simulink library "lib_FDM"  (R2019b)
settings: Solver=VariableStepAuto  StartTime=0.0  StopTime=10.0  RelTol=1e-3
values from neighbouring files (symbols this model uses):
  d = config.d_m    [computeTF.m]
undefined symbols (not defined in the file or in its folder): c_b_WGS, c_flat, c_grav, c_rot, c_rsma, Cd0, Cdcl, Cdcl2, Cl0, Cla, Cld, Cma, Cmd, Cmq, Cnb, Cnd, Cnr, Cra, Crd, Crp, Cy0, Cyb, Cyd, dmdt, Earth, HIL_Data, InitThrust, launchPos, me, mf, mp, Sref, tb, TF, theta0, WGS84
libraries: simulink_extras x14, $bdroot x7, simulink x5, lib_Fin_Deflections x3, aerolibasang x2, sharedtransform x1, aerolibtransform2 x1, aerolibbdyn x1, aerolibatmos2 x1, aerolibutil x1, aerolib6dof2 x1
(part 5 of 8)

== system lib_FDM/FDM/FDM_Sophisticated/stream_flow/calc_stream_flow/Subsystem1 ==
  vWEB : Inport
  vBEB : Inport  Port=2
  wBIB : Inport  Port=3
  rho : Inport  Port=4
  sos : Inport  Port=5
  AoA_Sideslip_Alphatot_Phi : Subsystem
      mask help:
      | Aus den Komponenten der Geschwindigkeit im ECEF-System, dargestellt im Body-System vBEB
      | werden Anstellwinkel (alpha), Schiebewinkel (beta), totaler Anstellwinkel (alpha_T) sowie Rollwinkel (phi) berechnet.
      | Die Ausgabe erfolgt als Bus in [rad]
      mask Help:
      | Name:
      | 
      |    AoA_sideslip_alphatot_phi
      | 
      | Beschreibung:
      | 
      |   Dieser Block berechnet Anstellwinkel, Schiebewinkel, totalen Anstellwinkel und Rollwinkel in [rad]
      |   aus der Geschwindigkeit vBEB (ECEF-System dargestellt in Body-Koordinaten)
      | 
      | Inputs   [dimension]  [data type] [unit]:
      | 
      |     vBEB    [3] [double] [m/s]
      | 
      | Outputs  [dimension]  [data type] [unit]:
      | 
      | aero_angle_bus [4] [bus] [-]
      |     alpha     [1] [double] [rad]
      |     beta       [1] [double] [rad]
      |     alpha_T [1] [double] [rad]
      |     phi         [1] [double] [rad]
      mask Display:
      | %port_label('input', 1, 'vBEB')
      | %port_label('output', 1, 'aero_angles')
      | disp('vBEB \rightarrow \alpha \beta \alpha_T \phi','texmode','on')
  Bus Selector : BusSelector  OutputSignals=al,be,th,fi
  Constant : Constant  Value=0.5
  Divide : Product  Inputs=*/
  Math Function1 : Math  Operator=square  SaturateOnIntegerOverflow=on
  Product1 : Product  Inputs=3
  Subtract : Sum  Inputs=+-
  calc_nondimensional_rates : Subsystem
  norm_of_vector : Subsystem
      mask help: computes the norm of a vector
      mask Help:
      | Name:
      | 
      |     norm_of_vector
      | 
      | Description:
      | 
      |     This block computes the L2-norm (length) of a vector.
      | 
      | Inputs  [size] [data type] [unit]:
      | 
      |     vector  [3] [double] [-]
      | 
      | Outputs  [size] [data type] [unit]:
      | 
      |     norm of vector  [1] [double] [-]
      mask Display: disp (' norm(r) ')
  al : Outport  VectorParamsAs1DForOutWhenUnconnected=off
  be : Outport  Port=2  VectorParamsAs1DForOutWhenUnconnected=off
  qdynB : Outport  Port=3  VectorParamsAs1DForOutWhenUnconnected=off
  MaB : Outport  Port=4  VectorParamsAs1DForOutWhenUnconnected=off
  a_vB : Outport  Port=5  VectorParamsAs1DForOutWhenUnconnected=off
  wBIB_star : Outport  Port=6  VectorParamsAs1DForOutWhenUnconnected=off
  th : Outport  Port=7  VectorParamsAs1DForOutWhenUnconnected=off
  fi : Outport  Port=8  VectorParamsAs1DForOutWhenUnconnected=off
  wires:
  Subtract/1 -> AoA_Sideslip_Alphatot_Phi/1(vBEB), norm_of_vector/1(vector)  "vBEB_a"
  vWEB/1 -> Subtract/2
  Bus Selector/4 -> fi/1  "<fi>"
  Bus Selector/3 -> th/1  "<th>"
  calc_nondimensional_rates/1(wBIB_star) -> wBIB_star/1
  wBIB/1 -> calc_nondimensional_rates/2(wBIB)
  Bus Selector/1 -> al/1  "<al>"
  rho/1 -> Product1/3
  Bus Selector/2 -> be/1  "<be>"
  Divide/1 -> MaB/1  "MaB"
  Constant/1 -> Product1/2
  Math Function1/1 -> Product1/1
  Product1/1 -> qdynB/1  "qdynB"
  norm_of_vector/1(norm_of_vector) -> Divide/1, a_vB/1, calc_nondimensional_rates/1(a_vB), Math Function1/1  "a_vB"
  vBEB/1 -> Subtract/1
  AoA_Sideslip_Alphatot_Phi/1(aero_angles) -> Bus Selector/1
  sos/1 -> Divide/2

== system lib_FDM/FDM/FDM_Sophisticated/stream_flow/calc_stream_flow/velocity_vector_transformation ==
  wIEE : Inport
  TIE : Inport  Port=2
  vBII : Inport  Port=3
  pBII : Inport  Port=4
  Add : Sum  Inputs=+-
  Product : Product  Multiplication=Matrix(*)
  cross_product : Subsystem
      mask help: cross product r3 = r1 x r2
      mask Help:
      | Name:
      | 
      |     cross_product
      | 
      | Description:
      | 
      |     This block implements the cross product r3 = r1 x r2.
      | 
      | Inputs  [size] [data type] [unit]:
      | 
      |     vector 1  [3] [double] [-]
      |     vector 2  [3] [double] [-]
      | 
      | Outputs  [size] [data type] [unit]:
      | 
      |     resulting vector  [3] [double] [-]
      mask Display: disp(' r3 = r1 x r2')
  vBEI : Outport  VectorParamsAs1DForOutWhenUnconnected=off
  wires:
  Add/1 -> vBEI/1  "vBEI"
  vBII/1 -> Add/1
  cross_product/1(r1_x_r2) -> Add/2  "de_vBEI"
  pBII/1 -> cross_product/2(r2)
  Product/1 -> cross_product/1(r1)  "wIEI"
  wIEE/1 -> Product/2
  TIE/1 -> Product/1

== system lib_FDM/FDM/FDM_Sophisticated/tmp/weather/atm_dynamic ==
  Add : Sum
  Add1 : Sum
  Bus Creator : BusCreator  Inputs=1
  Constant1 : Constant  Value=0
  Vector Concatenate : Concatenate  NumInputs=3
  course_angle_uncertainty : Constant  Value=HIL_Data.FDM.soph.bus1.unc_chW_bl
  course_angle_wind : Constant  Value=HIL_Data.FDM.soph.bus2.chW
  trafo_around_z_axis : Subsystem  mask(Transformation um z-Achse){}
      mask help: Dieser Block transformiert einen Vektor vec1 durch eine Drehung des Referenzkoordinatensystems um die z-Achse und um den Winkel gamma (in rad) in den Vektor vec2
      mask Help:
      | Name:
      | 
      |    trafo_around_z_axis
      | 
      | Beschreibung:
      | 
      |    Dieser Block transformiert einen Vektor vec1 durch eine Drehung des
      |    Referenzkoordinatensystems um die z-Achse und um den Winkel gamma
      |    (in rad) in den Vektor vec2
      | 
      | Inputs   [dimension]  [data type] [unit]:
      | 
      |     vec1    [3] [double] [-]
      |     gamma   [1] [double] [rad]
      | 
      | Outputs  [dimension]  [data type] [unit]:
      | 
      |     vec2  [3] [double] [-]
  vWW : Constant  Value=HIL_Data.FDM.soph.bus2.a_vBEW
  vWW_uncertainty : Constant  Value=HIL_Data.FDM.soph.bus1.unc_a_vBEW_bl
  vWEG : Outport  VectorParamsAs1DForOutWhenUnconnected=off
  wires:
  course_angle_wind/1 -> Add/1
  vWW_uncertainty/1 -> Add1/1
  Add/1 -> trafo_around_z_axis/2(gamma)
  Vector Concatenate/1 -> trafo_around_z_axis/1(vec1)
  vWW/1 -> Add1/2
  Constant1/1 -> Vector Concatenate/3, Vector Concatenate/2
  course_angle_uncertainty/1 -> Add/2
  Add1/1 -> Vector Concatenate/1
  trafo_around_z_axis/1(vec2) -> Bus Creator/1  "vWEG"
  Bus Creator/1 -> vWEG/1  "atm_dyn_bus"

== system lib_FDM/FDM/FDM_Sophisticated/weight_and_balance/d_moi/vector2diagonal_matrix ==
  vector : Inport
  Constant6 : Constant  Value=0
  Demux : Demux  Outputs=3
  Vector Concatenate1 : Concatenate  NumInputs=3
  Vector Concatenate2 : Concatenate  NumInputs=3
  Vector Concatenate3 : Concatenate  NumInputs=3
  Vector Concatenate4 : Concatenate  NumInputs=3  Mode=Multidimensional array  ConcatenateDimension=2
  diagonal_matrix : Outport  VectorParamsAs1DForOutWhenUnconnected=off
  wires:
  Demux/3 -> Vector Concatenate3/3
  Vector Concatenate3/1 -> Vector Concatenate4/3
  Vector Concatenate1/1 -> Vector Concatenate4/1
  Vector Concatenate2/1 -> Vector Concatenate4/2
  Demux/2 -> Vector Concatenate2/2
  Vector Concatenate4/1 -> diagonal_matrix/1
  Constant6/1 -> Vector Concatenate1/2, Vector Concatenate1/3, Vector Concatenate2/1, Vector Concatenate2/3, Vector Concatenate3/1, Vector Concatenate3/2
  vector/1 -> Demux/1
  Demux/1 -> Vector Concatenate1/1

== system lib_FDM/FDM/FDM_Sophisticated/weight_and_balance/moi/JMMM_linear_interpolation ==
  mM : Inport
  Constant16 : Constant  Value=HIL_Data.FDM.soph.bus1.JMMM_0
  Constant17 : Constant  Value=HIL_Data.FDM.soph.bus1.JMMM_e
  Constant18 : Constant  Value=HIL_Data.FDM.soph.bus1.mM_0
  Constant19 : Constant  Value=HIL_Data.FDM.soph.bus1.mM_e
  Constant20 : Constant  Value=HIL_Data.FDM.soph.bus1.mM_0
  Constant21 : Constant  Value=HIL_Data.FDM.soph.bus1.JMMM_0
  Divide : Product  Inputs=**/
  Subtract : Sum  Inputs=+-
  Subtract4 : Sum  Inputs=+-
  Subtract5 : Sum  Inputs=+-
  Subtract6 : Sum
  JMMM : Outport  VectorParamsAs1DForOutWhenUnconnected=off
  wires:
  Divide/1 -> Subtract6/2
  Constant21/1 -> Subtract6/1
  Subtract6/1 -> JMMM/1  "JMMM"
  Subtract4/1 -> Divide/3
  Subtract/1 -> Divide/2
  Constant16/1 -> Subtract/2
  Constant17/1 -> Subtract/1
  Constant18/1 -> Subtract4/2
  Constant19/1 -> Subtract4/1
  Constant20/1 -> Subtract5/2
  Subtract5/1 -> Divide/1
  mM/1 -> Subtract5/1

== system lib_FDM/FDM/FDM_Sophisticated/weight_and_balance/moi/moi_coordinate_transformation ==
  JMMM : Inport
  3_rot_mat : Subsystem  mask(Rotation um 1, 2 oder 3 Achsen){rot_1=Rotation um z-Achse, rot_2=Rotation um y-Achse, rot_3=Rotation um x-Achse}
      mask prompts: rot_1 "1. Rotation"; rot_2 "2. Rotation"; rot_3 "3. Rotation"
      mask help:
      | Dieser Block liefert die Rotationsmatrix T12 für den Fall zurück, dass sich das Ziel-Koordinatensystem (1) durch Drehungen um 1, 2 oder 3 Achsen gegenüber dem Ausgangskoordinatensystem (2) beschreiben lässt (passive Drehung).
      |
      | Die Anzahl der Rotation sowie die Reihenfolge ist frei einstellbar.
      |
      | Die Rotationswinkel haben die Einheit [rad].
      mask TypeOptions rot_1: Rotation um x-Achse | Rotation um y-Achse | Rotation um z-Achse
      mask TypeOptions rot_2: Rotation um x-Achse | Rotation um y-Achse | Rotation um z-Achse
      mask TypeOptions rot_3: Rotation um x-Achse | Rotation um y-Achse | Rotation um z-Achse
  Math Function : Math  Operator=transpose  SaturateOnIntegerOverflow=on
  Matrix Multiply : Product  Multiplication=Matrix(*)
  Matrix Multiply1 : Product  Multiplication=Matrix(*)
  Thrust_rot_z : Constant  Value=HIL_Data.FDM.soph.bus1.unc_prp_z
  thrust_rot_x : Constant  Value=HIL_Data.FDM.soph.bus1.unc_prp_x
  thrust_rot_y : Constant  Value=HIL_Data.FDM.soph.bus1.unc_prp_y
  JMMB : Outport  VectorParamsAs1DForOutWhenUnconnected=off
  wires:
  Thrust_rot_z/1 -> 3_rot_mat/1(wi1)
  thrust_rot_x/1 -> 3_rot_mat/3(wi3)
  thrust_rot_y/1 -> 3_rot_mat/2(wi2)
  Matrix Multiply1/1 -> JMMB/1  "JMMB"
  3_rot_mat/1(T12) -> Matrix Multiply/1, Math Function/1
  JMMM/1 -> Matrix Multiply/2
  Matrix Multiply/1 -> Matrix Multiply1/1
  Math Function/1 -> Matrix Multiply1/2

== system lib_FDM/FDM/FDM_Sophisticated/weight_and_balance/moi/moi_uncertainty ==
  JBBB_c : Inport
  Add7 : Sum
  Constant16 : Constant  Value=[HIL_Data.FDM.soph.bus1.unc_moi_Jxx,0,0;0,HIL_Data.FDM.soph.bus1.unc_moi_Jyy,0;0,0,HIL_Data.FDM.soph.bus1.unc_moi_Jzz]
  JBBB : Outport  VectorParamsAs1DForOutWhenUnconnected=off
  wires:
  Constant16/1 -> Add7/2
  JBBB_c/1 -> Add7/1
  Add7/1 -> JBBB/1  "JBBB"

== system lib_FDM/FDM/FDM_Sophisticated/weight_and_balance/moi/steiners_theorem_missile ==
  pBPB : Inport
  Constant : Constant  Value=HIL_Data.FDM.soph.bus1.mB_0
  Constant17 : Constant  Value=HIL_Data.FDM.soph.bus1.p0PB
  Product : Product
  Subtract : Sum  Inputs=+-
  create_deviation_matrix : Subsystem
  J_deviation : Outport  VectorParamsAs1DForOutWhenUnconnected=off
  wires:
  Constant/1 -> Product/1
  Subtract/1 -> create_deviation_matrix/1(pBXB)  "pB0B"
  Constant17/1 -> Subtract/2
  create_deviation_matrix/1(T_deviation) -> Product/2
  Product/1 -> J_deviation/1
  pBPB/1 -> Subtract/1

== system lib_FDM/FDM/FDM_Sophisticated/weight_and_balance/moi/steiners_theorem_motor ==
  pBPB : Inport
  mM : Inport  Port=2
  Constant16 : Constant  Value=HIL_Data.FDM.soph.bus1.pMPB
  Product : Product
  Subtract4 : Sum  Inputs=+-
  create_deviation_matrix1 : Subsystem
  JM_deviation : Outport  VectorParamsAs1DForOutWhenUnconnected=off
  wires:
  mM/1 -> Product/2
  Subtract4/1 -> create_deviation_matrix1/1(pBXB)  "pBMB"
  Constant16/1 -> Subtract4/2
  create_deviation_matrix1/1(T_deviation) -> Product/1
  pBPB/1 -> Subtract4/1
  Product/1 -> JM_deviation/1

== system lib_FDM/FDM/FDM_Student/Aerodynamics/-/Calc Thrust ==
  time : Inport
  If : If  IfExpression=u1<=2
  If Action Subsystem : Subsystem  TreatAsAtomicUnit=on
  If Action Subsystem1 : Subsystem  TreatAsAtomicUnit=on
  Merge : Merge
  Thrust : Outport  VectorParamsAs1DForOutWhenUnconnected=off
  wires:
  If/2 -> If Action Subsystem1/Action
  time/1 -> If/1
  Merge/1 -> Thrust/1
  If Action Subsystem1/1(Thrust1) -> Merge/2
  If/1 -> If Action Subsystem/Action
  If Action Subsystem/1(Thrust) -> Merge/1

== system lib_FDM/FDM/FDM_Student/Aerodynamics/Force Calc/CD_Wind ==
  CL : Inport
  CY : Inport  Port=2
  "C_D_0 " : Constant  Value=Cd0
  C_d_Cl : Gain  Gain=Cdcl
  C_d_Cl1 : Gain  Gain=Cdcl2
  C_d_Cl2 : Gain  Gain=Cdcl2
  C_d_Cl3 : Gain  Gain=Cdcl
  Square : Math  Operator=square  SaturateOnIntegerOverflow=on
  Square1 : Math  Operator=square  SaturateOnIntegerOverflow=on
  Sum1 : Sum  Inputs=|++
  Sum2 : Sum  Inputs=|+++
  Sum3 : Sum  Inputs=|++
  CD : Outport  VectorParamsAs1DForOutWhenUnconnected=off
  wires:
  C_d_Cl2/1 -> Sum2/1
  Square/1 -> C_d_Cl2/1
  CL/1 -> C_d_Cl/1, Square/1
  "C_D_0 "/1 -> Sum2/3
  C_d_Cl/1 -> Sum2/2
  CY/1 -> C_d_Cl3/1, Square1/1
  Square1/1 -> C_d_Cl1/1
  C_d_Cl1/1 -> Sum1/1
  C_d_Cl3/1 -> Sum1/2
  Sum2/1 -> Sum3/1  "CD"
  Sum1/1 -> Sum3/2
  Sum3/1 -> CD/1

== system lib_FDM/FDM/FDM_Student/Aerodynamics/Force Calc/CL_Wind ==
  AOA : Inport
  delta P : Inport  Port=2
  C_L_0 : Constant  Value=Cl0
  C_L_alpha : Gain  Gain=Cla
  C_L_delta : Gain  Gain=Cld
  Sum : Sum  Inputs=|+++
  CL : Outport  VectorParamsAs1DForOutWhenUnconnected=off
  wires:
  Sum/1 -> CL/1  "CL"
  AOA/1 -> C_L_alpha/1
  C_L_alpha/1 -> Sum/1
  C_L_delta/1 -> Sum/2
  delta P/1 -> C_L_delta/1
  C_L_0/1 -> Sum/3

== system lib_FDM/FDM/FDM_Student/Aerodynamics/Force Calc/CY_Wind ==
  beta : Inport
  delta Y : Inport  Port=2
  C_Y_0 : Constant  Value=Cy0
  C_y_beta : Gain  Gain=Cyb
  C_y_delta : Gain  Gain=Cyd
  Sum1 : Sum  Inputs=|+++
  Cy : Outport  VectorParamsAs1DForOutWhenUnconnected=off
  wires:
  beta/1 -> C_y_beta/1
  C_y_beta/1 -> Sum1/1
  C_y_delta/1 -> Sum1/2
  Sum1/1 -> Cy/1  "Cy"
  delta Y/1 -> C_y_delta/1
  C_Y_0/1 -> Sum1/3

== system lib_FDM/FDM/FDM_Student/Aerodynamics/Moment Calc/Calc CL Wind ==
  Vb : Inport
  w_Wind : Inport  Port=2
  delta R : Inport  Port=3
  AOA : Inport  Port=4
  Dot Product : DotProduct  InputSameDT=on  OutDataTypeStr=Inherit: Inherit via internal rule
  If : If  IfExpression=u1~=0
  If Action Subsystem : Subsystem  TreatAsAtomicUnit=on
  If Action Subsystem1 : Subsystem  TreatAsAtomicUnit=on
  Merge : Merge
  Sqrt : Sqrt  SaturateOnIntegerOverflow=on
  To Workspace : ToWorkspace  VariableName=Velocity  SampleTime=-1
      settings: Save2DSignal=2-D array (concatenate along first dimension)
  C_L : Outport  VectorParamsAs1DForOutWhenUnconnected=off
  wires:
  Dot Product/1 -> Sqrt/1
  Vb/1 -> Dot Product/1, Dot Product/2
  If/1 -> If Action Subsystem/Action
  Sqrt/1 -> To Workspace/1, If Action Subsystem/4(Vb), If/1
  If/2 -> If Action Subsystem1/Action
  Merge/1 -> C_L/1
  w_Wind/1 -> If Action Subsystem/1(w_Wind)
  delta R/1 -> If Action Subsystem/2(delta R)
  AOA/1 -> If Action Subsystem/3(AOA)
  If Action Subsystem1/1(CL) -> Merge/2
  If Action Subsystem/1(CL) -> Merge/1

== system lib_FDM/FDM/FDM_Student/Aerodynamics/Moment Calc/Calc CM Wind ==
  Vb : Inport
  alpha : Inport  Port=2
  delta p : Inport  Port=3
  w_Wind : Inport  Port=4
  Dot Product : DotProduct  InputSameDT=on  OutDataTypeStr=Inherit: Inherit via internal rule
  If Action Subsystem2 : Subsystem  TreatAsAtomicUnit=on
  If Action Subsystem3 : Subsystem  TreatAsAtomicUnit=on
  If1 : If  IfExpression=u1~=0
  Merge : Merge
  Sqrt : Sqrt  SaturateOnIntegerOverflow=on
  CM : Outport  VectorParamsAs1DForOutWhenUnconnected=off
  wires:
  Dot Product/1 -> Sqrt/1
  Sqrt/1 -> If Action Subsystem2/4(Vb), If1/1
  Vb/1 -> Dot Product/1, Dot Product/2
  If1/1 -> If Action Subsystem2/Action
  If1/2 -> If Action Subsystem3/Action
  If Action Subsystem2/1(CM) -> Merge/1
  If Action Subsystem3/1(CM) -> Merge/2
  Merge/1 -> CM/1
  alpha/1 -> If Action Subsystem2/1(alpha)
  delta p/1 -> If Action Subsystem2/2(delta p)
  w_Wind/1 -> If Action Subsystem2/3(w_Wind)

== system lib_FDM/FDM/FDM_Student/Aerodynamics/Moment Calc/Calc CN Wind ==
  Vb : Inport
  beta : Inport  Port=2
  delta Y : Inport  Port=3
  w_Wind : Inport  Port=4
  Dot Product : DotProduct  InputSameDT=on  OutDataTypeStr=Inherit: Inherit via internal rule
  If Action Subsystem2 : Subsystem  TreatAsAtomicUnit=on
  If Action Subsystem3 : Subsystem  TreatAsAtomicUnit=on
  If1 : If  IfExpression=u1~=0
  Merge : Merge
  Sqrt : Sqrt  SaturateOnIntegerOverflow=on
  CN : Outport  VectorParamsAs1DForOutWhenUnconnected=off
  wires:
  Dot Product/1 -> Sqrt/1
  Vb/1 -> Dot Product/2, Dot Product/1
  If1/1 -> If Action Subsystem2/Action
  If1/2 -> If Action Subsystem3/Action
  beta/1 -> If Action Subsystem2/1(beta)
  delta Y/1 -> If Action Subsystem2/2(delta Y)
  w_Wind/1 -> If Action Subsystem2/3(w_Wind)
  Sqrt/1 -> If Action Subsystem2/4(Vb), If1/1
  If Action Subsystem2/1(CN) -> Merge/1
  If Action Subsystem3/1(CN) -> Merge/2
  Merge/1 -> CN/1

== system lib_FDM/FDM/FDM_Student/Global Calculations/Calculate AOA, Sideslip and Airspeed/If Action Subsystem ==
  In1 : Inport
  Action Port : ActionPort
  "Incidence, Sideslip, & Airspeed" : aerolibasang/Incidence, Sideslip, & Airspeed
      settings: SourceProductName=Aerospace Blockset
  Mux : Mux  Inputs=3
  Out1 : Outport  VectorParamsAs1DForOutWhenUnconnected=off
  wires:
  In1/1 -> "Incidence, Sideslip, & Airspeed"/1
  "Incidence, Sideslip, & Airspeed"/3 -> Mux/3
  "Incidence, Sideslip, & Airspeed"/2 -> Mux/2
  "Incidence, Sideslip, & Airspeed"/1 -> Mux/1
  Mux/1 -> Out1/1

== system lib_FDM/FDM/FDM_Student/Global Calculations/Calculate AOA, Sideslip and Airspeed/If Action Subsystem1 ==
  In1 : Inport
  Action Port : ActionPort
  Mux : Mux  Inputs=3
  case1 : MATLAB Function  TreatAsAtomicUnit=on
  Out1 : Outport  VectorParamsAs1DForOutWhenUnconnected=off
  wires:
  In1/1 -> case1/1(Vb)
  case1/1(alpha) -> Mux/1
  case1/3(V) -> Mux/3
  case1/2(beta) -> Mux/2
  Mux/1 -> Out1/1

== system lib_FDM/FDM/FDM_Sophisticated/aerodynamics/aerodynamic_via_lookup/calc_aero_for_mom/cross_product ==
  note: Inputs [size]:
      |
      | r1 [3x1]
      | r2 [3x1]
  note: Outputs [size]:
      |
      | r1 x r2  [3x1]
  r1 : Inport
  r2 : Inport  Port=2
  Demux2 : Demux  Outputs=[1;1;1]
  Demux3 : Demux  Outputs=[1;1;1]
  Product{2..7} (6 alike) : Product  SaturateOnIntegerOverflow=on  RndMeth=Zero  InputSameDT=on  OutDataTypeStr=Inherit: Same as first input
  Reshape{,1..5} (6 alike) : Reshape  OutputDimensionality=Customize  OutputDimensions=1
  Sum : Sum  Inputs=+-  SaturateOnIntegerOverflow=on  InputSameDT=on  OutDataTypeStr=Inherit: Same as first input
  Sum1 : Sum  Inputs=+-  SaturateOnIntegerOverflow=on  InputSameDT=on  OutDataTypeStr=Inherit: Same as first input
  Sum2 : Sum  Inputs=+-  SaturateOnIntegerOverflow=on  InputSameDT=on  OutDataTypeStr=Inherit: Same as first input
  Vector Concatenate : Concatenate  NumInputs=3  Mode=Multidimensional array
  r1_x_r2 : Outport  PortDimensions=[3,1]  VectorParamsAs1DForOutWhenUnconnected=off
  wires:
  Vector Concatenate/1 -> r1_x_r2/1
  r2/1 -> Demux3/1
  r1/1 -> Demux2/1
  Sum2/1 -> Vector Concatenate/3
  Sum1/1 -> Vector Concatenate/2
  Sum/1 -> Vector Concatenate/1
  Product7/1 -> Sum2/2
  Product6/1 -> Sum2/1
  Product5/1 -> Sum1/2
  Product4/1 -> Sum1/1
  Product3/1 -> Sum/2
  Product2/1 -> Sum/1
  Demux3/1 -> Reshape3/1
  Demux2/3 -> Reshape2/1
  Demux3/2 -> Reshape4/1
  Demux3/3 -> Reshape5/1
  Demux2/2 -> Reshape1/1
  Demux2/1 -> Reshape/1
  Reshape/1 -> Product5/1, Product6/1
  Reshape1/1 -> Product7/1, Product2/1
  Reshape2/1 -> Product4/1, Product3/1
  Reshape3/1 -> Product4/2, Product7/2
  Reshape4/1 -> Product3/2, Product6/2
  Reshape5/1 -> Product2/2, Product5/2

== system lib_FDM/FDM/FDM_Sophisticated/aerodynamics/aerodynamic_via_lookup/calc_aero_for_mom/launch_rail ==
  hBE : Inport
  FBAB_c : Inport  Port=2
  Constant1 : Constant  Value=HIL_Data.FDM.soph.bus2.flag_I_aero_switch
  Constant3 : Constant  Value=0
  Subtract : Sum  Inputs=++-
  Switch : Switch  Criteria=u2 > Threshold  Threshold=0.05
  Vector Concatenate : Concatenate  NumInputs=3
  initial_altitude : Subsystem
  FBAB : Outport  VectorParamsAs1DForOutWhenUnconnected=off
  wires:
  initial_altitude/1(hBE_0) -> Subtract/3
  FBAB_c/1 -> Switch/1
  Vector Concatenate/1 -> Switch/3
  Switch/1 -> FBAB/1  "FBAB"
  Constant3/1 -> Vector Concatenate/3, Vector Concatenate/2, Vector Concatenate/1
  Subtract/1 -> Switch/2
  hBE/1 -> Subtract/1
  Constant1/1 -> Subtract/2

== system lib_FDM/FDM/FDM_Sophisticated/aerodynamics/aerodynamic_via_lookup/calc_aero_for_mom/launch_rail1 ==
  hBE : Inport
  MBAB_c : Inport  Port=2
  Constant1 : Constant  Value=HIL_Data.FDM.soph.bus2.flag_I_aero_switch
  Constant3 : Constant  Value=0
  Subtract : Sum  Inputs=++-
  Switch : Switch  Criteria=u2 > Threshold  Threshold=0.05
  Vector Concatenate : Concatenate  NumInputs=3
  initial_altitude : Subsystem
  MBAB : Outport  VectorParamsAs1DForOutWhenUnconnected=off
  wires:
  Constant1/1 -> Subtract/2
  hBE/1 -> Subtract/1
  Subtract/1 -> Switch/2
  Constant3/1 -> Vector Concatenate/1, Vector Concatenate/2, Vector Concatenate/3
  Switch/1 -> MBAB/1  "MBAB"
  Vector Concatenate/1 -> Switch/3
  MBAB_c/1 -> Switch/1
  initial_altitude/1(hBE_0) -> Subtract/3

== system lib_FDM/FDM/FDM_Sophisticated/aerodynamics/aerodynamic_via_lookup/calc_derivatives/Cl_derivatives_lookup ==
  aero_pre_lookup : Inport
  Bus Creator1 : BusCreator  Inputs=7
  Bus Selector2 : BusSelector  OutputSignals=k_Mach,f_Mach,k_alB,f_alB,k_beB,f_beB
  Cl_Interpolation : Interpolation_n-D  NumberOfTableDimensions=3  Table=HIL_Data.FDM.soph.bus1.aero.Cl  ExtrapMethod=Clip  DiagnosticForOutOfRangeInput=Warning  InternalRulePriority=Speed
      settings: InputPortMap=u0,u1,u2,u3,u4,u5
  Cl_delta_l_Interpolation : Interpolation_n-D  NumberOfTableDimensions=3  Table=HIL_Data.FDM.soph.bus1.aero.Cl_delta_l  ExtrapMethod=Clip  DiagnosticForOutOfRangeInput=Warning  InternalRulePriority=Speed
      settings: InputPortMap=u0,u1,u2,u3,u4,u5
  Cl_delta_m_Interpolation : Interpolation_n-D  NumberOfTableDimensions=3  Table=HIL_Data.FDM.soph.bus1.aero.Cl_delta_m  ExtrapMethod=Clip  DiagnosticForOutOfRangeInput=Warning  InternalRulePriority=Speed
      settings: InputPortMap=u0,u1,u2,u3,u4,u5
  Cl_delta_n_Interpolation : Interpolation_n-D  NumberOfTableDimensions=3  Table=HIL_Data.FDM.soph.bus1.aero.Cl_delta_n  ExtrapMethod=Clip  DiagnosticForOutOfRangeInput=Warning  InternalRulePriority=Speed
      settings: InputPortMap=u0,u1,u2,u3,u4,u5
  Clp_Interpolation : Interpolation_n-D  NumberOfTableDimensions=3  Table=HIL_Data.FDM.soph.bus1.aero.Clp  ExtrapMethod=Clip  DiagnosticForOutOfRangeInput=Warning  InternalRulePriority=Speed
      settings: InputPortMap=u0,u1,u2,u3,u4,u5
  Clq_Interpolation : Interpolation_n-D  NumberOfTableDimensions=3  Table=HIL_Data.FDM.soph.bus1.aero.Clq  ExtrapMethod=Clip  DiagnosticForOutOfRangeInput=Warning  InternalRulePriority=Speed
      settings: InputPortMap=u0,u1,u2,u3,u4,u5
  Clr_Interpolation : Interpolation_n-D  NumberOfTableDimensions=3  Table=HIL_Data.FDM.soph.bus1.aero.Clr  ExtrapMethod=Clip  DiagnosticForOutOfRangeInput=Warning  InternalRulePriority=Speed
      settings: InputPortMap=u0,u1,u2,u3,u4,u5
  Constant : Constant  Value=HIL_Data.FDM.soph.bus1.unc_aero_Cl_scale
  Product : Product
  Cl_deriv : Outport  VectorParamsAs1DForOutWhenUnconnected=off
  wires:
  Product/1 -> Bus Creator1/1  "Cl"
  Constant/1 -> Product/1
  Bus Creator1/1 -> Cl_deriv/1  "Cl_deriv_bus"
  Clp_Interpolation/1 -> Bus Creator1/2  "Clp"
  Cl_delta_l_Interpolation/1 -> Bus Creator1/5  "Cldl"
  aero_pre_lookup/1 -> Bus Selector2/1
  Cl_Interpolation/1 -> Product/2  "Cl"
  Cl_delta_m_Interpolation/1 -> Bus Creator1/6  "Cldm"
  Clr_Interpolation/1 -> Bus Creator1/4  "Clr"
  Clq_Interpolation/1 -> Bus Creator1/3  "Clq"
  Cl_delta_n_Interpolation/1 -> Bus Creator1/7  "Cldn"
  Bus Selector2/5 -> Cl_Interpolation/5, Clp_Interpolation/5, Clq_Interpolation/5, Clr_Interpolation/5, Cl_delta_l_Interpolation/5, Cl_delta_m_Interpolation/5, Cl_delta_n_Interpolation/5  "<k_beB>"
  Bus Selector2/1 -> Cl_Interpolation/1, Clp_Interpolation/1, Clq_Interpolation/1, Clr_Interpolation/1, Cl_delta_l_Interpolation/1, Cl_delta_m_Interpolation/1, Cl_delta_n_Interpolation/1  "<k_Mach>"
  Bus Selector2/2 -> Cl_Interpolation/2, Clp_Interpolation/2, Clq_Interpolation/2, Clr_Interpolation/2, Cl_delta_l_Interpolation/2, Cl_delta_m_Interpolation/2, Cl_delta_n_Interpolation/2  "<f_Mach>"
  Bus Selector2/3 -> Cl_Interpolation/3, Clp_Interpolation/3, Clq_Interpolation/3, Clr_Interpolation/3, Cl_delta_l_Interpolation/3, Cl_delta_m_Interpolation/3, Cl_delta_n_Interpolation/3  "<k_alB>"
  Bus Selector2/4 -> Cl_Interpolation/4, Clp_Interpolation/4, Clq_Interpolation/4, Clr_Interpolation/4, Cl_delta_l_Interpolation/4, Cl_delta_m_Interpolation/4, Cl_delta_n_Interpolation/4  "<f_alB>"
  Bus Selector2/6 -> Cl_Interpolation/6, Clp_Interpolation/6, Clq_Interpolation/6, Clr_Interpolation/6, Cl_delta_l_Interpolation/6, Cl_delta_m_Interpolation/6, Cl_delta_n_Interpolation/6  "<f_beB>"

== system lib_FDM/FDM/FDM_Sophisticated/aerodynamics/aerodynamic_via_lookup/calc_derivatives/Cm_derivatives_lookup ==
  aero_pre_lookup : Inport
  Bus Creator1 : BusCreator  Inputs=7
  Bus Selector2 : BusSelector  OutputSignals=k_Mach,f_Mach,k_alB,f_alB,k_beB,f_beB
  Cm_Interpolation : Interpolation_n-D  NumberOfTableDimensions=3  Table=HIL_Data.FDM.soph.bus1.aero.Cm  ExtrapMethod=Clip  DiagnosticForOutOfRangeInput=Warning  InternalRulePriority=Speed
      settings: InputPortMap=u0,u1,u2,u3,u4,u5
  Cm_delta_l_Interpolation : Interpolation_n-D  NumberOfTableDimensions=3  Table=HIL_Data.FDM.soph.bus1.aero.Cm_delta_l  ExtrapMethod=Clip  DiagnosticForOutOfRangeInput=Warning  InternalRulePriority=Speed
      settings: InputPortMap=u0,u1,u2,u3,u4,u5
  Cm_delta_m_Interpolation : Interpolation_n-D  NumberOfTableDimensions=3  Table=HIL_Data.FDM.soph.bus1.aero.Cm_delta_m  ExtrapMethod=Clip  DiagnosticForOutOfRangeInput=Warning  InternalRulePriority=Speed
      settings: InputPortMap=u0,u1,u2,u3,u4,u5
  Cm_delta_n_Interpolation : Interpolation_n-D  NumberOfTableDimensions=3  Table=HIL_Data.FDM.soph.bus1.aero.Cm_delta_n  ExtrapMethod=Clip  DiagnosticForOutOfRangeInput=Warning  InternalRulePriority=Speed
      settings: InputPortMap=u0,u1,u2,u3,u4,u5
  Cmp_Interpolation : Interpolation_n-D  NumberOfTableDimensions=3  Table=HIL_Data.FDM.soph.bus1.aero.Cmp  ExtrapMethod=Clip  DiagnosticForOutOfRangeInput=Warning  InternalRulePriority=Speed
      settings: InputPortMap=u0,u1,u2,u3,u4,u5
  Cmq_Interpolation : Interpolation_n-D  NumberOfTableDimensions=3  Table=HIL_Data.FDM.soph.bus1.aero.Cmq  ExtrapMethod=Clip  DiagnosticForOutOfRangeInput=Warning  InternalRulePriority=Speed
      settings: InputPortMap=u0,u1,u2,u3,u4,u5
  Cmr_Interpolation : Interpolation_n-D  NumberOfTableDimensions=3  Table=HIL_Data.FDM.soph.bus1.aero.Cmr  ExtrapMethod=Clip  DiagnosticForOutOfRangeInput=Warning  InternalRulePriority=Speed
      settings: InputPortMap=u0,u1,u2,u3,u4,u5
  Constant : Constant  Value=HIL_Data.FDM.soph.bus1.unc_aero_Cm_scale
  Product : Product
  Cm_deriv : Outport  VectorParamsAs1DForOutWhenUnconnected=off
  wires:
  Product/1 -> Bus Creator1/1  "Cm"
  Constant/1 -> Product/1
  Bus Selector2/4 -> Cm_Interpolation/4, Cmp_Interpolation/4, Cmq_Interpolation/4, Cmr_Interpolation/4, Cm_delta_l_Interpolation/4, Cm_delta_m_Interpolation/4, Cm_delta_n_Interpolation/4  "<f_alB>"
  Bus Selector2/3 -> Cm_Interpolation/3, Cmp_Interpolation/3, Cmq_Interpolation/3, Cmr_Interpolation/3, Cm_delta_l_Interpolation/3, Cm_delta_m_Interpolation/3, Cm_delta_n_Interpolation/3  "<k_alB>"
  Bus Selector2/2 -> Cm_Interpolation/2, Cmp_Interpolation/2, Cmq_Interpolation/2, Cmr_Interpolation/2, Cm_delta_l_Interpolation/2, Cm_delta_m_Interpolation/2, Cm_delta_n_Interpolation/2  "<f_Mach>"
  Bus Selector2/1 -> Cm_Interpolation/1, Cmp_Interpolation/1, Cmq_Interpolation/1, Cmr_Interpolation/1, Cm_delta_l_Interpolation/1, Cm_delta_m_Interpolation/1, Cm_delta_n_Interpolation/1  "<k_Mach>"
  Bus Selector2/6 -> Cm_Interpolation/6, Cmp_Interpolation/6, Cmq_Interpolation/6, Cmr_Interpolation/6, Cm_delta_l_Interpolation/6, Cm_delta_m_Interpolation/6, Cm_delta_n_Interpolation/6  "<f_beB>"
  aero_pre_lookup/1 -> Bus Selector2/1
  Cmp_Interpolation/1 -> Bus Creator1/2  "Cmp"
  Cm_delta_l_Interpolation/1 -> Bus Creator1/5  "Cmdl"
  Bus Selector2/5 -> Cm_Interpolation/5, Cmp_Interpolation/5, Cmq_Interpolation/5, Cmr_Interpolation/5, Cm_delta_l_Interpolation/5, Cm_delta_m_Interpolation/5, Cm_delta_n_Interpolation/5  "<k_beB>"
  Cmq_Interpolation/1 -> Bus Creator1/3  "Cmq"
  Cm_Interpolation/1 -> Product/2  "Cm"
  Cm_delta_n_Interpolation/1 -> Bus Creator1/7  "Cmdn"
  Cm_delta_m_Interpolation/1 -> Bus Creator1/6  "Cmdm"
  Cmr_Interpolation/1 -> Bus Creator1/4  "Cmr"
  Bus Creator1/1 -> Cm_deriv/1  "Cm_deriv_bus"

== system lib_FDM/FDM/FDM_Sophisticated/aerodynamics/aerodynamic_via_lookup/calc_derivatives/Cn_derivatives_lookup ==
  aero_pre_lookup : Inport
  Bus Creator1 : BusCreator  Inputs=7
  Bus Selector1 : BusSelector  OutputSignals=k_Mach,f_Mach,k_alB,f_alB,k_beB,f_beB
  Cn_Interpolation : Interpolation_n-D  NumberOfTableDimensions=3  Table=HIL_Data.FDM.soph.bus1.aero.Cn  ExtrapMethod=Clip  DiagnosticForOutOfRangeInput=Warning  InternalRulePriority=Speed
      settings: InputPortMap=u0,u1,u2,u3,u4,u5
  Cn_delta_l_Interpolation : Interpolation_n-D  NumberOfTableDimensions=3  Table=HIL_Data.FDM.soph.bus1.aero.Cn_delta_l  ExtrapMethod=Clip  DiagnosticForOutOfRangeInput=Warning  InternalRulePriority=Speed
      settings: InputPortMap=u0,u1,u2,u3,u4,u5
  Cn_delta_m_Interpolation : Interpolation_n-D  NumberOfTableDimensions=3  Table=HIL_Data.FDM.soph.bus1.aero.Cn_delta_m  ExtrapMethod=Clip  DiagnosticForOutOfRangeInput=Warning  InternalRulePriority=Speed
      settings: InputPortMap=u0,u1,u2,u3,u4,u5
  Cn_delta_n_Interpolation : Interpolation_n-D  NumberOfTableDimensions=3  Table=HIL_Data.FDM.soph.bus1.aero.Cn_delta_n  ExtrapMethod=Clip  DiagnosticForOutOfRangeInput=Warning  InternalRulePriority=Speed
      settings: InputPortMap=u0,u1,u2,u3,u4,u5
  Cnp_Interpolation : Interpolation_n-D  NumberOfTableDimensions=3  Table=HIL_Data.FDM.soph.bus1.aero.Cnp  ExtrapMethod=Clip  DiagnosticForOutOfRangeInput=Warning  InternalRulePriority=Speed
      settings: InputPortMap=u0,u1,u2,u3,u4,u5
  Cnq_Interpolation : Interpolation_n-D  NumberOfTableDimensions=3  Table=HIL_Data.FDM.soph.bus1.aero.Cnq  ExtrapMethod=Clip  DiagnosticForOutOfRangeInput=Warning  InternalRulePriority=Speed
      settings: InputPortMap=u0,u1,u2,u3,u4,u5
  Cnr_Interpolation : Interpolation_n-D  NumberOfTableDimensions=3  Table=HIL_Data.FDM.soph.bus1.aero.Cnr  ExtrapMethod=Clip  DiagnosticForOutOfRangeInput=Warning  InternalRulePriority=Speed
      settings: InputPortMap=u0,u1,u2,u3,u4,u5
  Constant : Constant  Value=HIL_Data.FDM.soph.bus1.unc_aero_Cn_scale
  Product : Product
  Cn_deriv : Outport  VectorParamsAs1DForOutWhenUnconnected=off
  wires:
  Product/1 -> Bus Creator1/1  "Cn"
  Constant/1 -> Product/1
  Bus Selector1/6 -> Cn_Interpolation/6, Cnp_Interpolation/6, Cnq_Interpolation/6, Cnr_Interpolation/6, Cn_delta_l_Interpolation/6, Cn_delta_m_Interpolation/6, Cn_delta_n_Interpolation/6  "<f_beB>"
  Cn_delta_l_Interpolation/1 -> Bus Creator1/5  "Cndl"
  Cn_delta_n_Interpolation/1 -> Bus Creator1/7  "Cndn"
  Cn_Interpolation/1 -> Product/2  "Cn"
  Cn_delta_m_Interpolation/1 -> Bus Creator1/6  "Cndm"
  Cnq_Interpolation/1 -> Bus Creator1/3  "Cnq"
  Cnr_Interpolation/1 -> Bus Creator1/4  "Cnr"
  Bus Selector1/5 -> Cn_Interpolation/5, Cnp_Interpolation/5, Cnq_Interpolation/5, Cnr_Interpolation/5, Cn_delta_l_Interpolation/5, Cn_delta_m_Interpolation/5, Cn_delta_n_Interpolation/5  "<k_beB>"
  Bus Creator1/1 -> Cn_deriv/1  "Cn_deriv_bus"
  Cnp_Interpolation/1 -> Bus Creator1/2  "Cnp"
  aero_pre_lookup/1 -> Bus Selector1/1
  Bus Selector1/2 -> Cn_Interpolation/2, Cnp_Interpolation/2, Cnq_Interpolation/2, Cnr_Interpolation/2, Cn_delta_l_Interpolation/2, Cn_delta_m_Interpolation/2, Cn_delta_n_Interpolation/2  "<f_Mach>"
  Bus Selector1/1 -> Cn_Interpolation/1, Cnp_Interpolation/1, Cnq_Interpolation/1, Cnr_Interpolation/1, Cn_delta_l_Interpolation/1, Cn_delta_m_Interpolation/1, Cn_delta_n_Interpolation/1  "<k_Mach>"
  Bus Selector1/4 -> Cn_Interpolation/4, Cnp_Interpolation/4, Cnq_Interpolation/4, Cnr_Interpolation/4, Cn_delta_l_Interpolation/4, Cn_delta_m_Interpolation/4, Cn_delta_n_Interpolation/4  "<f_alB>"
  Bus Selector1/3 -> Cn_Interpolation/3, Cnp_Interpolation/3, Cnq_Interpolation/3, Cnr_Interpolation/3, Cn_delta_l_Interpolation/3, Cn_delta_m_Interpolation/3, Cn_delta_n_Interpolation/3  "<k_alB>"

== system lib_FDM/FDM/FDM_Sophisticated/aerodynamics/aerodynamic_via_lookup/calc_derivatives/Cx_derivatives_lookup ==
  delta_t : Inport
  hBE : Inport  Port=2
  aero_pre_lookup : Inport  Port=3
  Bus Creator1 : BusCreator  Inputs=10
  Bus Selector1 : BusSelector  OutputSignals=k_Mach,f_Mach,k_alB,f_alB,k_beB,f_beB
  Constant : Constant  Value=HIL_Data.FDM.soph.bus1.unc_aero_Cx_scale
  Cx_Interpolation : Interpolation_n-D  NumberOfTableDimensions=3  Table=HIL_Data.FDM.soph.bus1.aero.Cx  ExtrapMethod=Clip  InternalRulePriority=Speed
      settings: InputPortMap=u0,u1,u2,u3,u4,u5
  Cx_alt_Interpolation : Interpolation_n-D  NumberOfTableDimensions=3  Table=HIL_Data.FDM.soph.bus1.aero.Cx_alt  ExtrapMethod=Clip  InternalRulePriority=Speed
      settings: InputPortMap=u0,u1,u2,u3,u4,u5
  Cx_base_Interpolation : Interpolation_n-D  NumberOfTableDimensions=3  Table=HIL_Data.FDM.soph.bus1.aero.Cx_base  ExtrapMethod=Clip  InternalRulePriority=Speed
      settings: InputPortMap=u0,u1,u2,u3,u4,u5
  Cx_delta_l_Interpolation : Interpolation_n-D  NumberOfTableDimensions=3  Table=HIL_Data.FDM.soph.bus1.aero.Cx_delta_l  ExtrapMethod=Clip  InternalRulePriority=Speed
      settings: InputPortMap=u0,u1,u2,u3,u4,u5
  Cx_delta_m_Interpolation : Interpolation_n-D  NumberOfTableDimensions=3  Table=HIL_Data.FDM.soph.bus1.aero.Cx_delta_m  ExtrapMethod=Clip  InternalRulePriority=Speed
      settings: InputPortMap=u0,u1,u2,u3,u4,u5
  Cx_delta_n_Interpolation : Interpolation_n-D  NumberOfTableDimensions=3  Table=HIL_Data.FDM.soph.bus1.aero.Cx_delta_n  ExtrapMethod=Clip  InternalRulePriority=Speed
      settings: InputPortMap=u0,u1,u2,u3,u4,u5
  Cx_delta_t_Interpolation : Interpolation_n-D  NumberOfTableDimensions=3  Table=HIL_Data.FDM.soph.bus1.aero.Cx_delta_t  ExtrapMethod=Clip  InternalRulePriority=Speed
      settings: InputPortMap=u0,u1,u2,u3,u4,u5
  Cxp_Interpolation : Interpolation_n-D  NumberOfTableDimensions=3  Table=HIL_Data.FDM.soph.bus1.aero.Cxp  ExtrapMethod=Clip  InternalRulePriority=Speed
      settings: InputPortMap=u0,u1,u2,u3,u4,u5
  Cxq_Interpolation : Interpolation_n-D  NumberOfTableDimensions=3  Table=HIL_Data.FDM.soph.bus1.aero.Cxq  ExtrapMethod=Clip  InternalRulePriority=Speed
      settings: InputPortMap=u0,u1,u2,u3,u4,u5
  Cxr_Interpolation : Interpolation_n-D  NumberOfTableDimensions=3  Table=HIL_Data.FDM.soph.bus1.aero.Cxr  ExtrapMethod=Clip  InternalRulePriority=Speed
      settings: InputPortMap=u0,u1,u2,u3,u4,u5
  Prelookup_altitude : PreLookup  BreakpointsData=HIL_Data.FDM.soph.bus1.aero.hoehe
  Prelookup_delta_t : PreLookup  BreakpointsData=HIL_Data.FDM.soph.bus1.aero.delta_t
  Product : Product
  Cx_deriv : Outport  VectorParamsAs1DForOutWhenUnconnected=off
  wires:
  Constant/1 -> Product/1
  Product/1 -> Bus Creator1/1  "Cx"
  Cx_delta_n_Interpolation/1 -> Bus Creator1/7  "Cxdn"
  Cx_delta_m_Interpolation/1 -> Bus Creator1/6  "Cxdm"
  Cx_delta_l_Interpolation/1 -> Bus Creator1/5  "Cxdl"
  delta_t/1 -> Prelookup_delta_t/1
  Bus Creator1/1 -> Cx_deriv/1  "Cx_deriv_bus"
  Prelookup_altitude/2 -> Cx_alt_Interpolation/6
  Prelookup_altitude/1 -> Cx_alt_Interpolation/5
  hBE/1 -> Prelookup_altitude/1
  aero_pre_lookup/1 -> Bus Selector1/1
  Prelookup_delta_t/1 -> Cx_delta_t_Interpolation/5
  Bus Selector1/1 -> Cx_Interpolation/1, Cxp_Interpolation/1, Cxq_Interpolation/1, Cxr_Interpolation/1, Cx_delta_l_Interpolation/1, Cx_alt_Interpolation/1, Cx_delta_t_Interpolation/1, Cx_base_Interpolation/1, Cx_delta_n_Interpolation/1, Cx_delta_m_Interpolation/1  "<k_Mach>"
  Bus Selector1/2 -> Cx_Interpolation/2, Cxp_Interpolation/2, Cxq_Interpolation/2, Cxr_Interpolation/2, Cx_delta_l_Interpolation/2, Cx_base_Interpolation/2, Cx_alt_Interpolation/2, Cx_delta_t_Interpolation/2, Cx_delta_n_Interpolation/2, Cx_delta_m_Interpolation/2  "<f_Mach>"
  Prelookup_delta_t/2 -> Cx_delta_t_Interpolation/6
  Bus Selector1/3 -> Cx_Interpolation/3, Cxp_Interpolation/3, Cxq_Interpolation/3, Cxr_Interpolation/3, Cx_delta_l_Interpolation/3, Cx_alt_Interpolation/3, Cx_delta_t_Interpolation/3, Cx_base_Interpolation/3, Cx_delta_n_Interpolation/3, Cx_delta_m_Interpolation/3  "<k_alB>"
  Bus Selector1/6 -> Cxp_Interpolation/6, Cxq_Interpolation/6, Cxr_Interpolation/6, Cx_delta_l_Interpolation/6, Cx_base_Interpolation/6, Cx_delta_n_Interpolation/6, Cx_delta_m_Interpolation/6, Cx_Interpolation/6  "<f_beB>"
  Bus Selector1/4 -> Cx_Interpolation/4, Cxp_Interpolation/4, Cxq_Interpolation/4, Cxr_Interpolation/4, Cx_delta_l_Interpolation/4, Cx_alt_Interpolation/4, Cx_delta_t_Interpolation/4, Cx_base_Interpolation/4, Cx_delta_n_Interpolation/4, Cx_delta_m_Interpolation/4  "<f_alB>"
  Cxp_Interpolation/1 -> Bus Creator1/2  "Cxp"
  Cx_delta_t_Interpolation/1 -> Bus Creator1/10  "Cx_alB_t"
  Cxr_Interpolation/1 -> Bus Creator1/4  "Cxr"
  Cxq_Interpolation/1 -> Bus Creator1/3  "Cxq"
  Cx_base_Interpolation/1 -> Bus Creator1/8  "Cx_base"
  Cx_Interpolation/1 -> Product/2  "Cx"
  Cx_alt_Interpolation/1 -> Bus Creator1/9  "Cx_alt"
  Bus Selector1/5 -> Cxp_Interpolation/5, Cxq_Interpolation/5, Cxr_Interpolation/5, Cx_delta_l_Interpolation/5, Cx_base_Interpolation/5, Cx_delta_n_Interpolation/5, Cx_delta_m_Interpolation/5, Cx_Interpolation/5  "<k_beB>"

== system lib_FDM/FDM/FDM_Sophisticated/aerodynamics/aerodynamic_via_lookup/calc_derivatives/Cy_derivatives_lookup ==
  aero_pre_lookup : Inport
  Bus Creator1 : BusCreator  Inputs=7
  Bus Selector1 : BusSelector  OutputSignals=k_Mach,f_Mach,k_alB,f_alB,k_beB,f_beB
  Constant : Constant  Value=HIL_Data.FDM.soph.bus1.unc_aero_Cy_scale
  Cy_Interpolation : Interpolation_n-D  NumberOfTableDimensions=3  Table=HIL_Data.FDM.soph.bus1.aero.Cy  ExtrapMethod=Clip  InternalRulePriority=Speed
      settings: InputPortMap=u0,u1,u2,u3,u4,u5
  Cy_delta_l_Interpolation : Interpolation_n-D  NumberOfTableDimensions=3  Table=HIL_Data.FDM.soph.bus1.aero.Cy_delta_l  ExtrapMethod=Clip  InternalRulePriority=Speed
      settings: InputPortMap=u0,u1,u2,u3,u4,u5
  Cy_delta_m_Interpolation : Interpolation_n-D  NumberOfTableDimensions=3  Table=HIL_Data.FDM.soph.bus1.aero.Cy_delta_m  ExtrapMethod=Clip  InternalRulePriority=Speed
      settings: InputPortMap=u0,u1,u2,u3,u4,u5
  Cy_delta_n_Interpolation : Interpolation_n-D  NumberOfTableDimensions=3  Table=HIL_Data.FDM.soph.bus1.aero.Cy_delta_n  ExtrapMethod=Clip  InternalRulePriority=Speed
      settings: InputPortMap=u0,u1,u2,u3,u4,u5
  Cyp_Interpolation : Interpolation_n-D  NumberOfTableDimensions=3  Table=HIL_Data.FDM.soph.bus1.aero.Cyp  ExtrapMethod=Clip  InternalRulePriority=Speed
      settings: InputPortMap=u0,u1,u2,u3,u4,u5
  Cyq_Interpolation : Interpolation_n-D  NumberOfTableDimensions=3  Table=HIL_Data.FDM.soph.bus1.aero.Cyq  ExtrapMethod=Clip  InternalRulePriority=Speed
      settings: InputPortMap=u0,u1,u2,u3,u4,u5
  Cyr_Interpolation : Interpolation_n-D  NumberOfTableDimensions=3  Table=HIL_Data.FDM.soph.bus1.aero.Cyr  ExtrapMethod=Clip  InternalRulePriority=Speed
      settings: InputPortMap=u0,u1,u2,u3,u4,u5
  Product : Product
  Cy_deriv : Outport  VectorParamsAs1DForOutWhenUnconnected=off
  wires:
  Product/1 -> Bus Creator1/1  "Cy"
  Constant/1 -> Product/1
  Cyq_Interpolation/1 -> Bus Creator1/3  "Cyq"
  Cyr_Interpolation/1 -> Bus Creator1/4  "Cyr"
  Bus Creator1/1 -> Cy_deriv/1  "Cy_deriv_bus"
  Cy_delta_m_Interpolation/1 -> Bus Creator1/6  "Cydm"
  Cy_delta_l_Interpolation/1 -> Bus Creator1/5  "Cydl"
  Cyp_Interpolation/1 -> Bus Creator1/2  "Cyp"
  aero_pre_lookup/1 -> Bus Selector1/1
  Bus Selector1/2 -> Cy_Interpolation/2, Cyp_Interpolation/2, Cyq_Interpolation/2, Cyr_Interpolation/2, Cy_delta_l_Interpolation/2, Cy_delta_m_Interpolation/2, Cy_delta_n_Interpolation/2  "<f_Mach>"
  Bus Selector1/1 -> Cy_Interpolation/1, Cyp_Interpolation/1, Cyq_Interpolation/1, Cyr_Interpolation/1, Cy_delta_l_Interpolation/1, Cy_delta_m_Interpolation/1, Cy_delta_n_Interpolation/1  "<k_Mach>"
  Bus Selector1/3 -> Cy_Interpolation/3, Cyp_Interpolation/3, Cyq_Interpolation/3, Cyr_Interpolation/3, Cy_delta_l_Interpolation/3, Cy_delta_m_Interpolation/3, Cy_delta_n_Interpolation/3  "<k_alB>"
  Bus Selector1/4 -> Cy_Interpolation/4, Cyp_Interpolation/4, Cyq_Interpolation/4, Cyr_Interpolation/4, Cy_delta_l_Interpolation/4, Cy_delta_m_Interpolation/4, Cy_delta_n_Interpolation/4  "<f_alB>"
  Bus Selector1/6 -> Cy_Interpolation/6, Cyp_Interpolation/6, Cyq_Interpolation/6, Cyr_Interpolation/6, Cy_delta_l_Interpolation/6, Cy_delta_m_Interpolation/6, Cy_delta_n_Interpolation/6  "<f_beB>"
  Bus Selector1/5 -> Cy_Interpolation/5, Cyp_Interpolation/5, Cyq_Interpolation/5, Cyr_Interpolation/5, Cy_delta_l_Interpolation/5, Cy_delta_m_Interpolation/5, Cy_delta_n_Interpolation/5  "<k_beB>"
  Cy_delta_n_Interpolation/1 -> Bus Creator1/7  "Cydn"
  Cy_Interpolation/1 -> Product/2  "Cy"

== system lib_FDM/FDM/FDM_Sophisticated/aerodynamics/aerodynamic_via_lookup/calc_derivatives/Cz_derivatives_lookup ==
  aero_pre_lookup : Inport
  Bus Creator1 : BusCreator  Inputs=7
  Bus Selector2 : BusSelector  OutputSignals=k_Mach,f_Mach,k_alB,f_alB,k_beB,f_beB
  Constant : Constant  Value=HIL_Data.FDM.soph.bus1.unc_aero_Cz_scale
  Cz_Interpolation : Interpolation_n-D  NumberOfTableDimensions=3  Table=HIL_Data.FDM.soph.bus1.aero.Cz  ExtrapMethod=Clip  DiagnosticForOutOfRangeInput=Warning  InternalRulePriority=Speed
      settings: InputPortMap=u0,u1,u2,u3,u4,u5
  Cz_delta_l_Interpolation : Interpolation_n-D  NumberOfTableDimensions=3  Table=HIL_Data.FDM.soph.bus1.aero.Cz_delta_l  ExtrapMethod=Clip  DiagnosticForOutOfRangeInput=Warning  InternalRulePriority=Speed
      settings: InputPortMap=u0,u1,u2,u3,u4,u5
  Cz_delta_m_Interpolation : Interpolation_n-D  NumberOfTableDimensions=3  Table=HIL_Data.FDM.soph.bus1.aero.Cz_delta_m  ExtrapMethod=Clip  DiagnosticForOutOfRangeInput=Warning  InternalRulePriority=Speed
      settings: InputPortMap=u0,u1,u2,u3,u4,u5
  Cz_delta_n_Interpolation : Interpolation_n-D  NumberOfTableDimensions=3  Table=HIL_Data.FDM.soph.bus1.aero.Cz_delta_n  ExtrapMethod=Clip  DiagnosticForOutOfRangeInput=Warning  InternalRulePriority=Speed
      settings: InputPortMap=u0,u1,u2,u3,u4,u5
  Czp_Interpolation : Interpolation_n-D  NumberOfTableDimensions=3  Table=HIL_Data.FDM.soph.bus1.aero.Czp  ExtrapMethod=Clip  DiagnosticForOutOfRangeInput=Warning  InternalRulePriority=Speed
      settings: InputPortMap=u0,u1,u2,u3,u4,u5
  Czq_Interpolation : Interpolation_n-D  NumberOfTableDimensions=3  Table=HIL_Data.FDM.soph.bus1.aero.Czq  ExtrapMethod=Clip  DiagnosticForOutOfRangeInput=Warning  InternalRulePriority=Speed
      settings: InputPortMap=u0,u1,u2,u3,u4,u5
  Czr_Interpolation : Interpolation_n-D  NumberOfTableDimensions=3  Table=HIL_Data.FDM.soph.bus1.aero.Czr  ExtrapMethod=Clip  DiagnosticForOutOfRangeInput=Warning  InternalRulePriority=Speed
      settings: InputPortMap=u0,u1,u2,u3,u4,u5
  Product : Product
  Cz_deriv : Outport  VectorParamsAs1DForOutWhenUnconnected=off
  wires:
  Product/1 -> Bus Creator1/1  "Cz"
  Constant/1 -> Product/1
  Czr_Interpolation/1 -> Bus Creator1/4  "Czr"
  Czp_Interpolation/1 -> Bus Creator1/2  "Czp"
  aero_pre_lookup/1 -> Bus Selector2/1
  Czq_Interpolation/1 -> Bus Creator1/3  "Czq"
  Bus Creator1/1 -> Cz_deriv/1  "Cz_deriv_bus"
  Cz_delta_l_Interpolation/1 -> Bus Creator1/5  "Czdl"
  Cz_delta_n_Interpolation/1 -> Bus Creator1/7  "Czdn"
  Bus Selector2/3 -> Cz_Interpolation/3, Czp_Interpolation/3, Czq_Interpolation/3, Czr_Interpolation/3, Cz_delta_l_Interpolation/3, Cz_delta_m_Interpolation/3, Cz_delta_n_Interpolation/3  "<k_alB>"
  Bus Selector2/6 -> Cz_Interpolation/6, Czp_Interpolation/6, Czq_Interpolation/6, Czr_Interpolation/6, Cz_delta_l_Interpolation/6, Cz_delta_m_Interpolation/6, Cz_delta_n_Interpolation/6  "<f_beB>"
  Cz_delta_m_Interpolation/1 -> Bus Creator1/6  "Czdm"
  Cz_Interpolation/1 -> Product/2  "Cz"
  Bus Selector2/5 -> Cz_Interpolation/5, Czp_Interpolation/5, Czq_Interpolation/5, Czr_Interpolation/5, Cz_delta_l_Interpolation/5, Cz_delta_m_Interpolation/5, Cz_delta_n_Interpolation/5  "<k_beB>"
  Bus Selector2/1 -> Cz_Interpolation/1, Czp_Interpolation/1, Czq_Interpolation/1, Czr_Interpolation/1, Cz_delta_l_Interpolation/1, Cz_delta_m_Interpolation/1, Cz_delta_n_Interpolation/1  "<k_Mach>"
  Bus Selector2/2 -> Cz_Interpolation/2, Czp_Interpolation/2, Czq_Interpolation/2, Czr_Interpolation/2, Cz_delta_l_Interpolation/2, Cz_delta_m_Interpolation/2, Cz_delta_n_Interpolation/2  "<f_Mach>"
  Bus Selector2/4 -> Cz_Interpolation/4, Czp_Interpolation/4, Czq_Interpolation/4, Czr_Interpolation/4, Cz_delta_l_Interpolation/4, Cz_delta_m_Interpolation/4, Cz_delta_n_Interpolation/4  "<f_alB>"

== system lib_FDM/FDM/FDM_Sophisticated/aerodynamics/aerodynamic_via_lookup/calc_derivatives/aerodynamics_pre_lookup ==
  alB : Inport
  beB : Inport  Port=2
  Ma : Inport  Port=3
  Bus Creator1 : BusCreator  Inputs=6
  Prelookup_Mach : PreLookup  BreakpointsData=HIL_Data.FDM.soph.bus1.aero.Ma
  Prelookup_alB : PreLookup  BreakpointsData=HIL_Data.FDM.soph.bus1.aero.alpha
  Prelookup_beB : PreLookup  BreakpointsData=HIL_Data.FDM.soph.bus1.aero.beta
  aero_pre_lookup : Outport  VectorParamsAs1DForOutWhenUnconnected=off
  wires:
  beB/1 -> Prelookup_beB/1
  alB/1 -> Prelookup_alB/1
  Prelookup_beB/2 -> Bus Creator1/6  "f_beB"
  Prelookup_beB/1 -> Bus Creator1/5  "k_beB"
  Prelookup_Mach/1 -> Bus Creator1/1  "k_Mach"
  Prelookup_Mach/2 -> Bus Creator1/2  "f_Mach"
  Ma/1 -> Prelookup_Mach/1
  Prelookup_alB/2 -> Bus Creator1/4  "f_alB"
  Prelookup_alB/1 -> Bus Creator1/3  "k_alB"
  Bus Creator1/1 -> aero_pre_lookup/1  "aero_pre_lookup_bus"

== system lib_FDM/FDM/FDM_Sophisticated/aerodynamics/aerodynamic_via_lookup/calc_derivatives/calc_total_deflection_angle ==
  etB_deg : Inport
  zeB_deg : Inport  Port=2
  alB : Inport  Port=3
  beB : Inport  Port=4
  Abs : Abs
  Abs1 : Abs
  Abs2 : Abs
  Add : Sum
  Constant3 : Constant  Value=2
  Degrees to Radians : simulink_extras/Transformations/Degrees to Radians
  Degrees to Radians1 : simulink_extras/Transformations/Degrees to Radians
  Divide2 : Product  Inputs=**/
  Product1 : Product
  Product6 : Product
  Product7 : Product
  Radians to Degrees1 : simulink_extras/Transformations/Radians to Degrees
  Saturation : Saturate  UpperLimit=inf  LowerLimit=100*eps
      settings: AttributesFormatString=|
      | %<UpperLimit>
      | %<LowerLimit>
  Sqrt : Sqrt  SaturateOnIntegerOverflow=on
  Trigonometric Function : Trigonometry  Operator=acos
  Trigonometric Function1 : Trigonometry  Operator=cos
  Trigonometric Function2 : Trigonometry  Operator=cos
  delta_t : Outport  VectorParamsAs1DForOutWhenUnconnected=off
  wires:
  Radians to Degrees1/1 -> Saturation/1  "alB_t_deg"
  Trigonometric Function/1 -> Radians to Degrees1/1  "alB_t"
  Degrees to Radians1/1 -> Trigonometric Function2/1
  Degrees to Radians/1 -> Trigonometric Function1/1
  Abs2/1 -> delta_t/1  "delta_t"
  alB/1 -> Degrees to Radians/1, Abs/1
  Product1/1 -> Trigonometric Function/1
  Sqrt/1 -> Divide2/2
  Product7/1 -> Add/2
  beB/1 -> Degrees to Radians1/1, Abs1/1
  Add/1 -> Divide2/1
  Trigonometric Function1/1 -> Product1/1
  Constant3/1 -> Sqrt/1
  zeB_deg/1 -> Product7/2
  Abs/1 -> Product6/1
  etB_deg/1 -> Product6/2
  Trigonometric Function2/1 -> Product1/2
  Divide2/1 -> Abs2/1
  Abs1/1 -> Product7/1
  Saturation/1 -> Divide2/3
  Product6/1 -> Add/1

== system lib_FDM/FDM/FDM_Sophisticated/environment/WGS84_Gravitation/WGS84_2_ECEF/WGS84 Transformation Parameter  ==
  phi : Inport
  Add2 : Sum  Inputs=+-
  Divide : Product  Inputs=**
  Divide1 : Product  Inputs=**
  Divide2 : Product  Inputs=**
  Divide3 : Product  Inputs=/*
  Sqrt : Sqrt  SaturateOnIntegerOverflow=on
  Subsystem : Subsystem
  Trigonometric Function : Trigonometry
  "WGS84 Semi-major Axis, [m]" : Constant  Value=c_rsma
  "WGS84 Semi-minor Axis, [m]" : Constant  Value=c_b_WGS
  a3 : Constant
  N : Outport  VectorParamsAs1DForOutWhenUnconnected=off
  e : Outport  Port=2  VectorParamsAs1DForOutWhenUnconnected=off
  wires:
  phi/1 -> Trigonometric Function/1
  Add2/1 -> Sqrt/1
  Subsystem/1(e) -> Divide/1, Divide/2, e/1
  Divide/1 -> Divide2/2  "e^2"
  Trigonometric Function/1 -> Divide1/1, Divide1/2
  Divide2/1 -> Add2/2
  a3/1 -> Add2/1
  Sqrt/1 -> Divide3/1
  Divide3/1 -> N/1  "N"
  Divide1/1 -> Divide2/1  "sin(phi)^2"
  "WGS84 Semi-major Axis, [m]"/1 -> Divide3/2, Subsystem/2(a)  "c_rsma"
  "WGS84 Semi-minor Axis, [m]"/1 -> Subsystem/1(b)  "c_b_WGS"
